simulink model "control_base_ss"  (R2020a)
settings: Solver=VariableStepAuto  StartTime=0.0  StopTime=10  RelTol=1e-3
undefined symbols (not defined in the file or in its folder): C, k, kbb
libraries: simulink x1
settings Model: Creator=adpan  LastModifiedBy=adpan

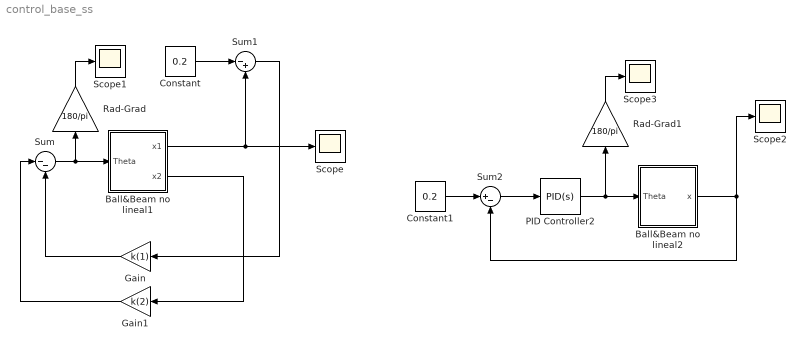
== system control_base_ss ==
  Ball&Beam no lineal1 : Subsystem
  Ball&Beam no lineal2 : Subsystem
  Constant : Constant  Value=0.2
  Constant1 : Constant  Value=0.2
  Gain : Gain  Gain=k(1)
  Gain1 : Gain  Gain=k(2)
  PID Controller2 : simulink/Continuous/PID Controller  Controller=PID  Form=Parallel  TimeDomain=Continuous-time  UseExternalTs=off  SampleTime=-1  IntegratorMethod=Forward Euler  FilterMethod=Forward Euler  ControllerParametersSource=internal  P=C.Kp  I=C.Ki  D=C.Kd  UseFilter=on  N=300  TunerSelectOption=Transfer Function Based (PID Tuner App)  InitialConditionSource=internal  InitialConditionForIntegrator=0  InitialConditionForFilter=0  DifferentiatorICPrevScaledInput=0  ExternalReset=none  TrackingMode=off  Kt=1  LimitOutput=off  UpperSaturationLimit=inf  LowerSaturationLimit=-inf  LinearizeAsGain=on  AntiWindupMode=none  Kb=1  POutMin=[]  POutMax=[]  IOutMin=[]  IOutMax=[]  DOutMin=[]  DOutMax=[]  NOutMin=[]  NOutMax=[]  SumOutMin=[]  SumOutMax=[]  SaturationOutMin=[]  SaturationOutMax=[]  PParamMin=[]  PParamMax=[]  IParamMin=[]  IParamMax=[]  DParamMin=[]  DParamMax=[]  NParamMin=[]  NParamMax=[]  KbParamMin=[]  KbParamMax=[]  KtParamMin=[]  KtParamMax=[]  KbOutMin=[]  KbOutMax=[]  KtOutMin=[]  KtOutMax=[]  IntegratorOutMin=[]  IntegratorOutMax=[]  FilterOutMin=[]  FilterOutMax=[]  SumI1OutMin=[]  SumI1OutMax=[]  SumI2OutMin=[]  SumI2OutMax=[]  SumI3OutMin=[]  SumI3OutMax=[]  SumI4OutMin=[]  SumI4OutMax=[]  SumDOutMin=[]  SumDOutMax=[]  DifferentiatorOutMin=[]  DifferentiatorOutMax=[]  FilterDiffOutCoefMin=[]  FilterDiffOutCoefMax=[]  ReciprocalOutMin=[]  ReciprocalOutMax=[]  SumDenOutMin=[]  SumDenOutMax=[]  SumNumOutMin=[]  SumNumOutMax=[]  DivideOutMin=[]  DivideOutMax=[]  UdiffTsProdOutMin=[]  UdiffTsProdOutMax=[]  NTsProdOutMin=[]  NTsProdOutMax=[]  UintegralTsProdOutMin=[]  UintegralTsProdOutMax=[]  UngainTsProdOutMin=[]  UngainTsProdOutMax=[]  IntegratorContinuousStateAttributes=''  IntegratorStateMustResolveToSignalObject=off  IntegratorRTWStateStorageClass=Auto  FilterContinuousStateAttributes=''  FilterStateMustResolveToSignalObject=off  FilterRTWStateStorageClass=Auto  ParallelPVariant=InternalParameters  IdealPVariant=Disabled  IVariant=InternalParameters  DVariant=InternalParameters  IntegratorVariant=Continuous  SatVariant=Disabled  AWVariant=Passthrough  PCopyVariant=Disabled  TRVariant=Disabled  FdbkBlocksVariant=Forward  IdealPFdbkVariant=Disabled  SatFdbkVariant=Disabled  DerivativeFilterVariant=ContFilter  NVariant=InternalParameters  NCopyVariant=Disabled  FilterICVariant=InternalICsFilter  IntegratorICVariant=InternalICs  ExternalResetVariant=Disabled  TRSumVariant=Passthrough  SumFdbkVariant=Disabled  SumVariant=Sum_PID  TsampFilterVariant=InternalTs  TsampNgainVariant=Passthrough  TsampIntegralVariant=Passthrough
  Rad-Grad : Gain  Gain=180/pi
  Rad-Grad1 : Gain  Gain=180/pi
  Scope{,1..3} (4 alike) : Scope
  Sum : Sum  Inputs=|--
  Sum1 : Sum  Inputs=|-+
  Sum2 : Sum  Inputs=|+-
  wires:
  Ball&Beam no lineal1/1(x1) -> Scope/1, Sum1/2
  Sum/1 -> Ball&Beam no lineal1/1(Theta), Rad-Grad/1
  Gain/1 -> Sum/2
  Gain1/1 -> Sum/1
  Sum1/1 -> Gain/1
  Ball&Beam no lineal1/2(x2) -> Gain1/1
  Constant/1 -> Sum1/1
  Ball&Beam no lineal2/1(x) -> Scope2/1, Sum2/2
  PID Controller2/1 -> Rad-Grad1/1, Ball&Beam no lineal2/1(Theta)
  Sum2/1 -> PID Controller2/1
  Constant1/1 -> Sum2/1
  Rad-Grad/1 -> Scope1/1
  Rad-Grad1/1 -> Scope3/1

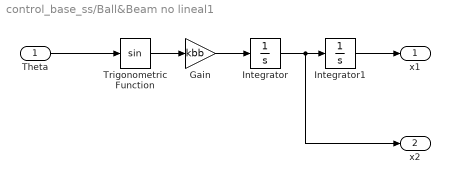
== system control_base_ss/Ball&Beam no lineal1 ==
  Theta : Inport
  Gain : Gain  Gain=kbb
  Integrator : Integrator
  Integrator1 : Integrator
  Trigonometric Function : Trigonometry
  x1 : Outport
  x2 : Outport  Port=2
  wires:
  Integrator/1 -> x2/1, Integrator1/1
  Integrator1/1 -> x1/1
  Gain/1 -> Integrator/1
  Trigonometric Function/1 -> Gain/1
  Theta/1 -> Trigonometric Function/1

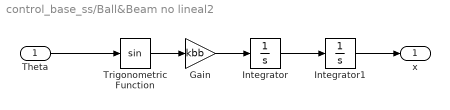
== system control_base_ss/Ball&Beam no lineal2 ==
  Theta : Inport
  Gain : Gain  Gain=kbb
  Integrator : Integrator
  Integrator1 : Integrator
  Trigonometric Function : Trigonometry
  x : Outport
  wires:
  Integrator/1 -> Integrator1/1
  Integrator1/1 -> x/1
  Gain/1 -> Integrator/1
  Trigonometric Function/1 -> Gain/1
  Theta/1 -> Trigonometric Function/1
